simulink model "TST_RailP_VD"  (R2016b)
settings: Solver=FixedStepDiscrete  StartTime=0.0  StopTime=simTime  FixedStep=sampleTime  RelTol=1e-3
values from neighbouring files (symbols this model uses):
  testCase = 1    [initTST_RailP_VD_001.m]    (also in initTST_RailP_VD_002.m = 2)
libraries: simulink x7, UnitTest_Lib x4
settings Model: Creator=liangyunbo  LastModifiedBy=liangyunbo
settings DebuggingCC: SignalRangeChecking=error

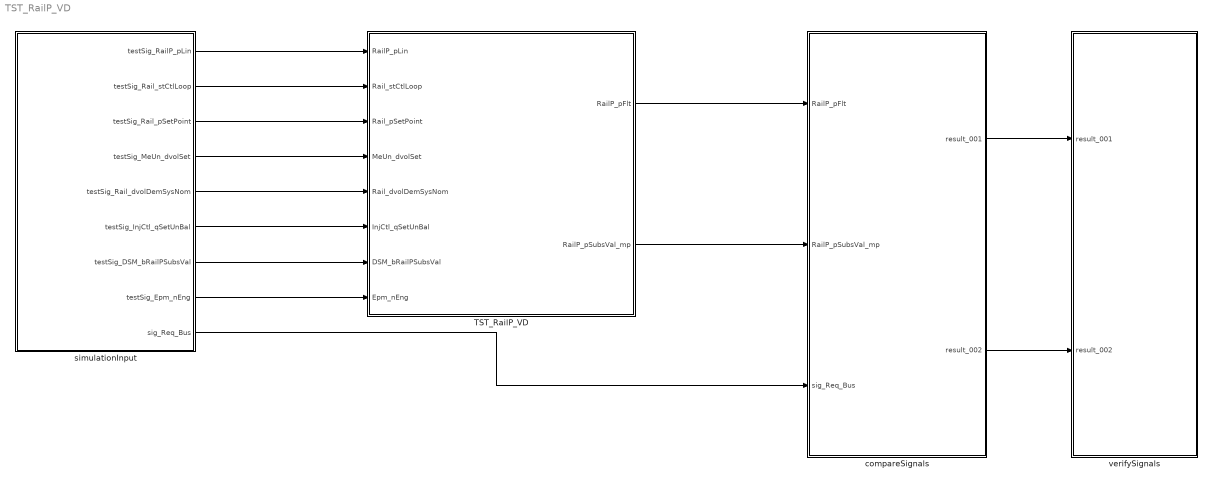
== system TST_RailP_VD ==
  TST_RailP_VD : Subsystem
  compareSignals : Subsystem
  simulationInput : Subsystem
  verifySignals : Subsystem
  wires:
  simulationInput/1(testSig_RailP_pLin) -> TST_RailP_VD/1(RailP_pLin)
  simulationInput/2(testSig_Rail_stCtlLoop) -> TST_RailP_VD/2(Rail_stCtlLoop)
  simulationInput/3(testSig_Rail_pSetPoint) -> TST_RailP_VD/3(Rail_pSetPoint)
  simulationInput/4(testSig_MeUn_dvolSet) -> TST_RailP_VD/4(MeUn_dvolSet)
  simulationInput/5(testSig_Rail_dvolDemSysNom) -> TST_RailP_VD/5(Rail_dvolDemSysNom)
  simulationInput/6(testSig_InjCtl_qSetUnBal) -> TST_RailP_VD/6(InjCtl_qSetUnBal)
  simulationInput/7(testSig_DSM_bRailPSubsVal) -> TST_RailP_VD/7(DSM_bRailPSubsVal)
  simulationInput/8(testSig_Epm_nEng) -> TST_RailP_VD/8(Epm_nEng)
  TST_RailP_VD/1(RailP_pFlt) -> compareSignals/1(RailP_pFlt)
  TST_RailP_VD/2(RailP_pSubsVal_mp) -> compareSignals/2(RailP_pSubsVal_mp)
  simulationInput/9(sig_Req_Bus) -> compareSignals/3(sig_Req_Bus)
  compareSignals/1(result_001) -> verifySignals/1(result_001)
  compareSignals/2(result_002) -> verifySignals/2(result_002)

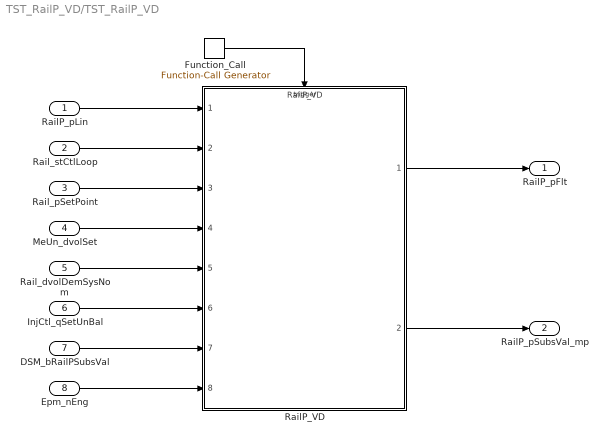
== system TST_RailP_VD/TST_RailP_VD ==
  RailP_pLin : Inport
  Rail_stCtlLoop : Inport  Port=2
  Rail_pSetPoint : Inport  Port=3
  MeUn_dvolSet : Inport  Port=4
  Rail_dvolDemSysNom : Inport  Port=5
  InjCtl_qSetUnBal : Inport  Port=6
  DSM_bRailPSubsVal : Inport  Port=7
  Epm_nEng : Inport  Port=8
  Function_Call : simulink/Ports & Subsystems/Function-Call Generator  sample_time=sampleTime  numberOfIterations=1
  RailP_VD : ModelReference  ModelNameDialog=RailP_VD  SimulationMode=Normal  ModelReferenceVersion=1.40  TriggerPortName=function  TriggerPortTriggerType=function-call  TriggerPortStatesWhenEnabling=held
  RailP_pFlt : Outport
  RailP_pSubsVal_mp : Outport  Port=2
  wires:
  Function_Call/1 -> RailP_VD/Trigger
  RailP_pLin/1 -> RailP_VD/1
  Rail_stCtlLoop/1 -> RailP_VD/2
  Rail_pSetPoint/1 -> RailP_VD/3
  MeUn_dvolSet/1 -> RailP_VD/4
  Rail_dvolDemSysNom/1 -> RailP_VD/5
  InjCtl_qSetUnBal/1 -> RailP_VD/6
  DSM_bRailPSubsVal/1 -> RailP_VD/7
  Epm_nEng/1 -> RailP_VD/8
  RailP_VD/1 -> RailP_pFlt/1
  RailP_VD/2 -> RailP_pSubsVal_mp/1

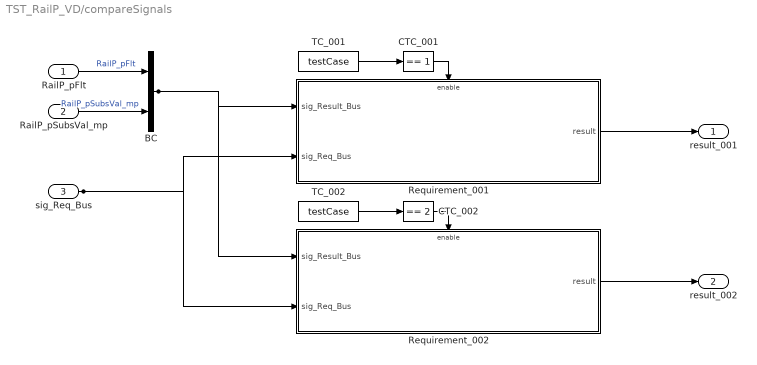
== system TST_RailP_VD/compareSignals ==
  RailP_pFlt : Inport
  RailP_pSubsVal_mp : Inport  Port=2
  sig_Req_Bus : Inport  Port=3
  BC : BusCreator  Inputs=2
  CTC_001 : simulink/Logic and Bit Operations/Compare To Constant  relop===  const=1  OutDataTypeStr=boolean
  CTC_002 : simulink/Logic and Bit Operations/Compare To Constant  relop===  const=2  OutDataTypeStr=boolean
  Requirement_001 : Subsystem
  Requirement_002 : Subsystem
  TC_001 : Constant  Value=testCase
  TC_002 : Constant  Value=testCase
  result_001 : Outport
  result_002 : Outport  Port=2
  wires:
  RailP_pFlt/1 -> BC/1  "RailP_pFlt"
  RailP_pSubsVal_mp/1 -> BC/2  "RailP_pSubsVal_mp"
  TC_001/1 -> CTC_001/1
  CTC_001/1 -> Requirement_001/Enable
  sig_Req_Bus/1 -> Requirement_001/2(sig_Req_Bus), Requirement_002/2(sig_Req_Bus)
  BC/1 -> Requirement_001/1(sig_Result_Bus), Requirement_002/1(sig_Result_Bus)
  Requirement_001/1(result) -> result_001/1
  TC_002/1 -> CTC_002/1
  CTC_002/1 -> Requirement_002/Enable
  Requirement_002/1(result) -> result_002/1

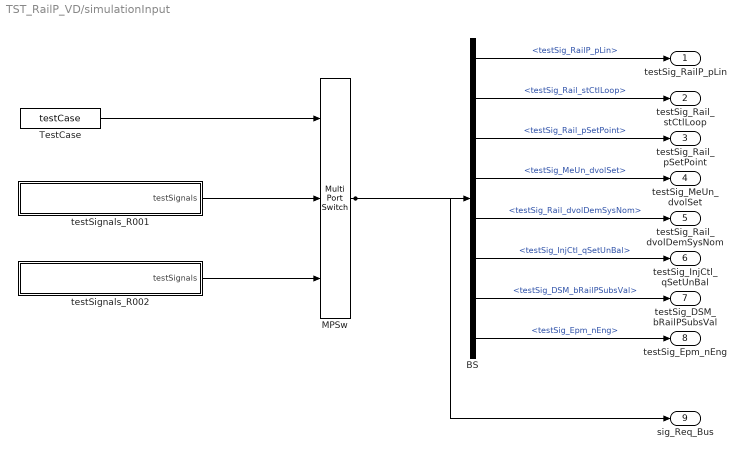
== system TST_RailP_VD/simulationInput ==
  BS : BusSelector  OutputSignals=testSig_RailP_pLin,testSig_Rail_stCtlLoop,testSig_Rail_pSetPoint,testSig_MeUn_dvolSet,testSig_Rail_dvolDemSysNom,testSig_InjCtl_qSetUnBal,testSig_DSM_bRailPSubsVal,testSig_Epm_nEng
  MPSw : MultiPortSwitch  Inputs=2  SaturateOnIntegerOverflow=on  InputSameDT=on
  TestCase : Constant  Value=testCase
  testSignals_R001 : Subsystem
  testSignals_R002 : Subsystem
  testSig_RailP_pLin : Outport
  testSig_Rail_stCtlLoop : Outport  Port=2
  testSig_Rail_pSetPoint : Outport  Port=3
  testSig_MeUn_dvolSet : Outport  Port=4
  testSig_Rail_dvolDemSysNom : Outport  Port=5
  testSig_InjCtl_qSetUnBal : Outport  Port=6
  testSig_DSM_bRailPSubsVal : Outport  Port=7
  testSig_Epm_nEng : Outport  Port=8
  sig_Req_Bus : Outport  Port=9
  wires:
  BS/1 -> testSig_RailP_pLin/1  "<testSig_RailP_pLin>"
  BS/2 -> testSig_Rail_stCtlLoop/1  "<testSig_Rail_stCtlLoop>"
  BS/3 -> testSig_Rail_pSetPoint/1  "<testSig_Rail_pSetPoint>"
  BS/4 -> testSig_MeUn_dvolSet/1  "<testSig_MeUn_dvolSet>"
  BS/5 -> testSig_Rail_dvolDemSysNom/1  "<testSig_Rail_dvolDemSysNom>"
  BS/6 -> testSig_InjCtl_qSetUnBal/1  "<testSig_InjCtl_qSetUnBal>"
  BS/7 -> testSig_DSM_bRailPSubsVal/1  "<testSig_DSM_bRailPSubsVal>"
  BS/8 -> testSig_Epm_nEng/1  "<testSig_Epm_nEng>"
  MPSw/1 -> BS/1, sig_Req_Bus/1
  TestCase/1 -> MPSw/1
  testSignals_R001/1(testSignals) -> MPSw/2
  testSignals_R002/1(testSignals) -> MPSw/3

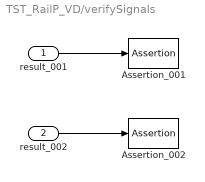
== system TST_RailP_VD/verifySignals ==
  result_001 : Inport
  result_002 : Inport  Port=2
  Assertion_001 : Assertion  Enabled=off
  Assertion_002 : Assertion  Enabled=off
  wires:
  result_001/1 -> Assertion_001/1
  result_002/1 -> Assertion_002/1

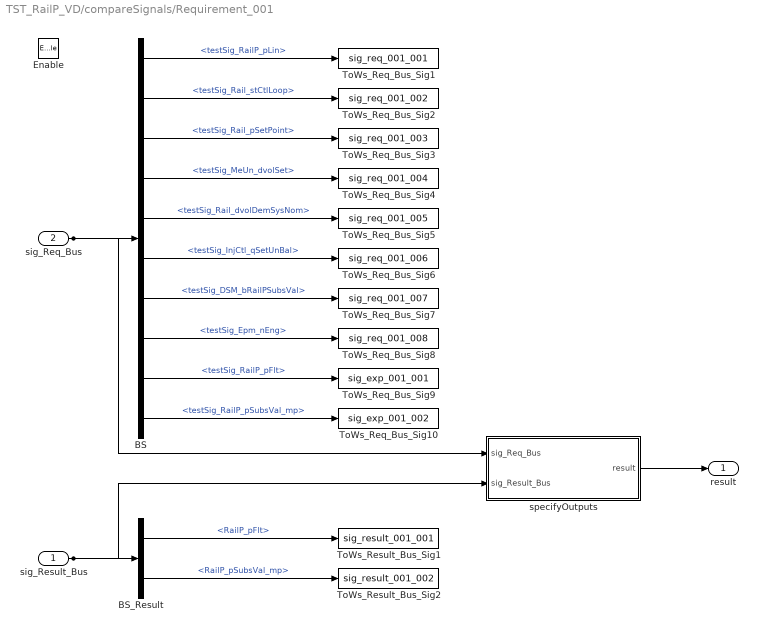
== system TST_RailP_VD/compareSignals/Requirement_001 ==
  sig_Result_Bus : Inport
  sig_Req_Bus : Inport  Port=2
  Enable : EnablePort
  BS : BusSelector  OutputSignals=testSig_RailP_pLin,testSig_Rail_stCtlLoop,testSig_Rail_pSetPoint,testSig_MeUn_dvolSet,testSig_Rail_dvolDemSysNom,testSig_InjCtl_qSetUnBal,testSig_DSM_bRailPSubsVal,testSig_Epm_nEng,testSig_RailP_pFlt,testSig_RailP_pSubsVal_mp
  BS_Result : BusSelector  OutputSignals=RailP_pFlt,RailP_pSubsVal_mp
  ToWs_Req_Bus_Sig1 : ToWorkspace  VariableName=sig_req_001_001  SaveFormat=Structure With Time
  ToWs_Req_Bus_Sig10 : ToWorkspace  VariableName=sig_exp_001_002  SaveFormat=Structure With Time
  ToWs_Req_Bus_Sig2 : ToWorkspace  VariableName=sig_req_001_002  SaveFormat=Structure With Time
  ToWs_Req_Bus_Sig3 : ToWorkspace  VariableName=sig_req_001_003  SaveFormat=Structure With Time
  ToWs_Req_Bus_Sig4 : ToWorkspace  VariableName=sig_req_001_004  SaveFormat=Structure With Time
  ToWs_Req_Bus_Sig5 : ToWorkspace  VariableName=sig_req_001_005  SaveFormat=Structure With Time
  ToWs_Req_Bus_Sig6 : ToWorkspace  VariableName=sig_req_001_006  SaveFormat=Structure With Time
  ToWs_Req_Bus_Sig7 : ToWorkspace  VariableName=sig_req_001_007  SaveFormat=Structure With Time
  ToWs_Req_Bus_Sig8 : ToWorkspace  VariableName=sig_req_001_008  SaveFormat=Structure With Time
  ToWs_Req_Bus_Sig9 : ToWorkspace  VariableName=sig_exp_001_001  SaveFormat=Structure With Time
  ToWs_Result_Bus_Sig1 : ToWorkspace  VariableName=sig_result_001_001  SaveFormat=Structure With Time
  ToWs_Result_Bus_Sig2 : ToWorkspace  VariableName=sig_result_001_002  SaveFormat=Structure With Time
  specifyOutputs : Subsystem
  result : Outport
  wires:
  sig_Req_Bus/1 -> BS/1, specifyOutputs/1(sig_Req_Bus)
  BS/1 -> ToWs_Req_Bus_Sig1/1  "<testSig_RailP_pLin>"
  BS/2 -> ToWs_Req_Bus_Sig2/1  "<testSig_Rail_stCtlLoop>"
  BS/3 -> ToWs_Req_Bus_Sig3/1  "<testSig_Rail_pSetPoint>"
  BS/4 -> ToWs_Req_Bus_Sig4/1  "<testSig_MeUn_dvolSet>"
  BS/5 -> ToWs_Req_Bus_Sig5/1  "<testSig_Rail_dvolDemSysNom>"
  BS/6 -> ToWs_Req_Bus_Sig6/1  "<testSig_InjCtl_qSetUnBal>"
  BS/7 -> ToWs_Req_Bus_Sig7/1  "<testSig_DSM_bRailPSubsVal>"
  BS/8 -> ToWs_Req_Bus_Sig8/1  "<testSig_Epm_nEng>"
  BS/9 -> ToWs_Req_Bus_Sig9/1  "<testSig_RailP_pFlt>"
  BS/10 -> ToWs_Req_Bus_Sig10/1  "<testSig_RailP_pSubsVal_mp>"
  sig_Result_Bus/1 -> BS_Result/1, specifyOutputs/2(sig_Result_Bus)
  BS_Result/1 -> ToWs_Result_Bus_Sig1/1  "<RailP_pFlt>"
  BS_Result/2 -> ToWs_Result_Bus_Sig2/1  "<RailP_pSubsVal_mp>"
  specifyOutputs/1(result) -> result/1

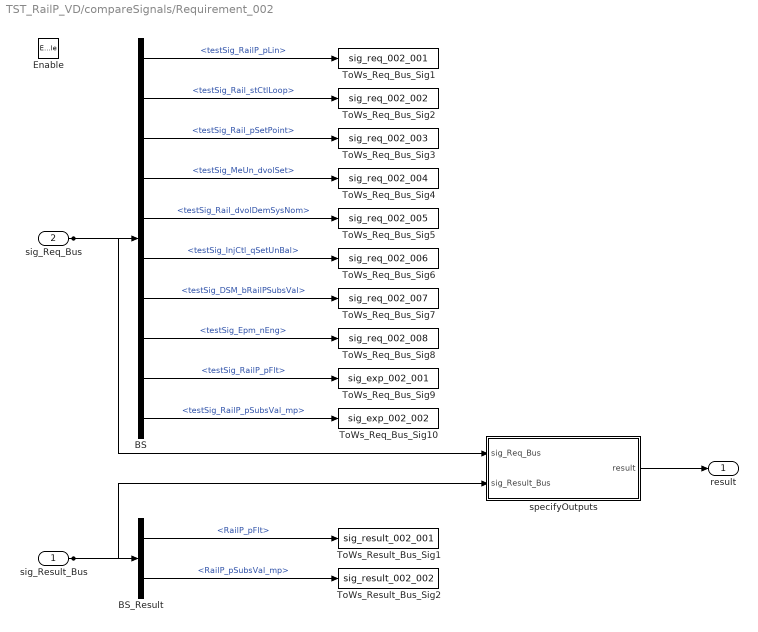
== system TST_RailP_VD/compareSignals/Requirement_002 ==
  sig_Result_Bus : Inport
  sig_Req_Bus : Inport  Port=2
  Enable : EnablePort
  BS : BusSelector  OutputSignals=testSig_RailP_pLin,testSig_Rail_stCtlLoop,testSig_Rail_pSetPoint,testSig_MeUn_dvolSet,testSig_Rail_dvolDemSysNom,testSig_InjCtl_qSetUnBal,testSig_DSM_bRailPSubsVal,testSig_Epm_nEng,testSig_RailP_pFlt,testSig_RailP_pSubsVal_mp
  BS_Result : BusSelector  OutputSignals=RailP_pFlt,RailP_pSubsVal_mp
  ToWs_Req_Bus_Sig1 : ToWorkspace  VariableName=sig_req_002_001  SaveFormat=Structure With Time
  ToWs_Req_Bus_Sig10 : ToWorkspace  VariableName=sig_exp_002_002  SaveFormat=Structure With Time
  ToWs_Req_Bus_Sig2 : ToWorkspace  VariableName=sig_req_002_002  SaveFormat=Structure With Time
  ToWs_Req_Bus_Sig3 : ToWorkspace  VariableName=sig_req_002_003  SaveFormat=Structure With Time
  ToWs_Req_Bus_Sig4 : ToWorkspace  VariableName=sig_req_002_004  SaveFormat=Structure With Time
  ToWs_Req_Bus_Sig5 : ToWorkspace  VariableName=sig_req_002_005  SaveFormat=Structure With Time
  ToWs_Req_Bus_Sig6 : ToWorkspace  VariableName=sig_req_002_006  SaveFormat=Structure With Time
  ToWs_Req_Bus_Sig7 : ToWorkspace  VariableName=sig_req_002_007  SaveFormat=Structure With Time
  ToWs_Req_Bus_Sig8 : ToWorkspace  VariableName=sig_req_002_008  SaveFormat=Structure With Time
  ToWs_Req_Bus_Sig9 : ToWorkspace  VariableName=sig_exp_002_001  SaveFormat=Structure With Time
  ToWs_Result_Bus_Sig1 : ToWorkspace  VariableName=sig_result_002_001  SaveFormat=Structure With Time
  ToWs_Result_Bus_Sig2 : ToWorkspace  VariableName=sig_result_002_002  SaveFormat=Structure With Time
  specifyOutputs : Subsystem
  result : Outport
  wires:
  sig_Req_Bus/1 -> BS/1, specifyOutputs/1(sig_Req_Bus)
  BS/1 -> ToWs_Req_Bus_Sig1/1  "<testSig_RailP_pLin>"
  BS/2 -> ToWs_Req_Bus_Sig2/1  "<testSig_Rail_stCtlLoop>"
  BS/3 -> ToWs_Req_Bus_Sig3/1  "<testSig_Rail_pSetPoint>"
  BS/4 -> ToWs_Req_Bus_Sig4/1  "<testSig_MeUn_dvolSet>"
  BS/5 -> ToWs_Req_Bus_Sig5/1  "<testSig_Rail_dvolDemSysNom>"
  BS/6 -> ToWs_Req_Bus_Sig6/1  "<testSig_InjCtl_qSetUnBal>"
  BS/7 -> ToWs_Req_Bus_Sig7/1  "<testSig_DSM_bRailPSubsVal>"
  BS/8 -> ToWs_Req_Bus_Sig8/1  "<testSig_Epm_nEng>"
  BS/9 -> ToWs_Req_Bus_Sig9/1  "<testSig_RailP_pFlt>"
  BS/10 -> ToWs_Req_Bus_Sig10/1  "<testSig_RailP_pSubsVal_mp>"
  sig_Result_Bus/1 -> BS_Result/1, specifyOutputs/2(sig_Result_Bus)
  BS_Result/1 -> ToWs_Result_Bus_Sig1/1  "<RailP_pFlt>"
  BS_Result/2 -> ToWs_Result_Bus_Sig2/1  "<RailP_pSubsVal_mp>"
  specifyOutputs/1(result) -> result/1

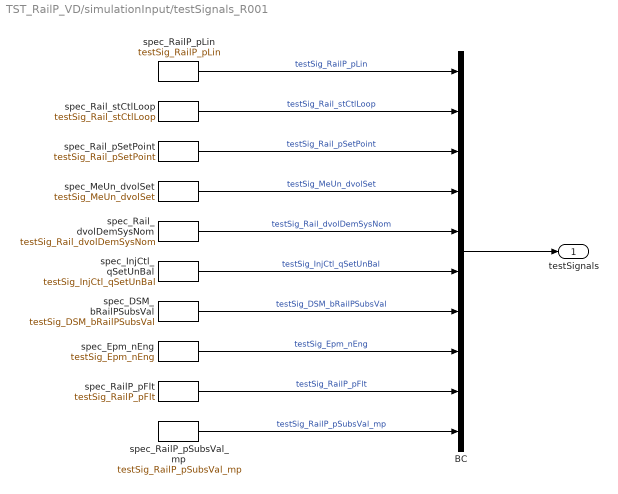
== system TST_RailP_VD/simulationInput/testSignals_R001 ==
  BC : BusCreator  Inputs=10
  spec_DSM_bRailPSubsVal : FromWorkspace  VariableName=testSig_DSM_bRailPSubsVal  Interpolate=off  OutputAfterFinalValue=Holding final value
  spec_Epm_nEng : FromWorkspace  VariableName=testSig_Epm_nEng  Interpolate=off  OutputAfterFinalValue=Holding final value
  spec_InjCtl_qSetUnBal : FromWorkspace  VariableName=testSig_InjCtl_qSetUnBal  Interpolate=off  OutputAfterFinalValue=Holding final value
  spec_MeUn_dvolSet : FromWorkspace  VariableName=testSig_MeUn_dvolSet  Interpolate=off  OutputAfterFinalValue=Holding final value
  spec_RailP_pFlt : FromWorkspace  VariableName=testSig_RailP_pFlt  Interpolate=off  OutputAfterFinalValue=Holding final value
  spec_RailP_pLin : FromWorkspace  VariableName=testSig_RailP_pLin  Interpolate=off  OutputAfterFinalValue=Holding final value
  spec_RailP_pSubsVal_mp : FromWorkspace  VariableName=testSig_RailP_pSubsVal_mp  Interpolate=off  OutputAfterFinalValue=Holding final value
  spec_Rail_dvolDemSysNom : FromWorkspace  VariableName=testSig_Rail_dvolDemSysNom  Interpolate=off  OutputAfterFinalValue=Holding final value
  spec_Rail_pSetPoint : FromWorkspace  VariableName=testSig_Rail_pSetPoint  Interpolate=off  OutputAfterFinalValue=Holding final value
  spec_Rail_stCtlLoop : FromWorkspace  VariableName=testSig_Rail_stCtlLoop  Interpolate=off  OutputAfterFinalValue=Holding final value
  testSignals : Outport
  wires:
  BC/1 -> testSignals/1
  spec_RailP_pLin/1 -> BC/1  "testSig_RailP_pLin"
  spec_Rail_stCtlLoop/1 -> BC/2  "testSig_Rail_stCtlLoop"
  spec_Rail_pSetPoint/1 -> BC/3  "testSig_Rail_pSetPoint"
  spec_MeUn_dvolSet/1 -> BC/4  "testSig_MeUn_dvolSet"
  spec_Rail_dvolDemSysNom/1 -> BC/5  "testSig_Rail_dvolDemSysNom"
  spec_InjCtl_qSetUnBal/1 -> BC/6  "testSig_InjCtl_qSetUnBal"
  spec_DSM_bRailPSubsVal/1 -> BC/7  "testSig_DSM_bRailPSubsVal"
  spec_Epm_nEng/1 -> BC/8  "testSig_Epm_nEng"
  spec_RailP_pFlt/1 -> BC/9  "testSig_RailP_pFlt"
  spec_RailP_pSubsVal_mp/1 -> BC/10  "testSig_RailP_pSubsVal_mp"

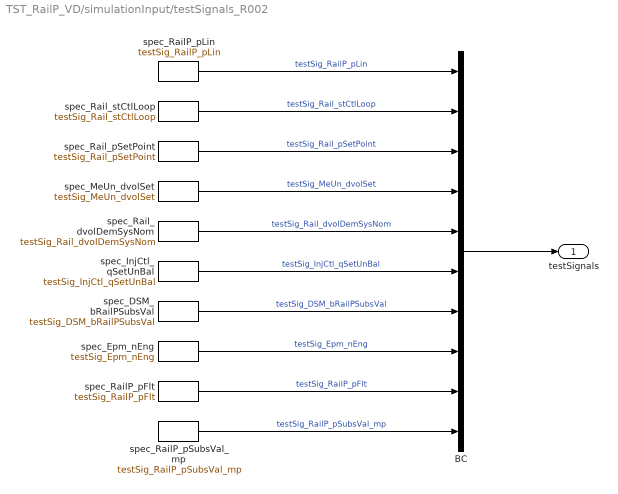
== system TST_RailP_VD/simulationInput/testSignals_R002 ==
  BC : BusCreator  Inputs=10
  spec_DSM_bRailPSubsVal : FromWorkspace  VariableName=testSig_DSM_bRailPSubsVal  Interpolate=off  OutputAfterFinalValue=Holding final value
  spec_Epm_nEng : FromWorkspace  VariableName=testSig_Epm_nEng  Interpolate=off  OutputAfterFinalValue=Holding final value
  spec_InjCtl_qSetUnBal : FromWorkspace  VariableName=testSig_InjCtl_qSetUnBal  Interpolate=off  OutputAfterFinalValue=Holding final value
  spec_MeUn_dvolSet : FromWorkspace  VariableName=testSig_MeUn_dvolSet  Interpolate=off  OutputAfterFinalValue=Holding final value
  spec_RailP_pFlt : FromWorkspace  VariableName=testSig_RailP_pFlt  Interpolate=off  OutputAfterFinalValue=Holding final value
  spec_RailP_pLin : FromWorkspace  VariableName=testSig_RailP_pLin  Interpolate=off  OutputAfterFinalValue=Holding final value
  spec_RailP_pSubsVal_mp : FromWorkspace  VariableName=testSig_RailP_pSubsVal_mp  Interpolate=off  OutputAfterFinalValue=Holding final value
  spec_Rail_dvolDemSysNom : FromWorkspace  VariableName=testSig_Rail_dvolDemSysNom  Interpolate=off  OutputAfterFinalValue=Holding final value
  spec_Rail_pSetPoint : FromWorkspace  VariableName=testSig_Rail_pSetPoint  Interpolate=off  OutputAfterFinalValue=Holding final value
  spec_Rail_stCtlLoop : FromWorkspace  VariableName=testSig_Rail_stCtlLoop  Interpolate=off  OutputAfterFinalValue=Holding final value
  testSignals : Outport
  wires:
  BC/1 -> testSignals/1
  spec_RailP_pLin/1 -> BC/1  "testSig_RailP_pLin"
  spec_Rail_stCtlLoop/1 -> BC/2  "testSig_Rail_stCtlLoop"
  spec_Rail_pSetPoint/1 -> BC/3  "testSig_Rail_pSetPoint"
  spec_MeUn_dvolSet/1 -> BC/4  "testSig_MeUn_dvolSet"
  spec_Rail_dvolDemSysNom/1 -> BC/5  "testSig_Rail_dvolDemSysNom"
  spec_InjCtl_qSetUnBal/1 -> BC/6  "testSig_InjCtl_qSetUnBal"
  spec_DSM_bRailPSubsVal/1 -> BC/7  "testSig_DSM_bRailPSubsVal"
  spec_Epm_nEng/1 -> BC/8  "testSig_Epm_nEng"
  spec_RailP_pFlt/1 -> BC/9  "testSig_RailP_pFlt"
  spec_RailP_pSubsVal_mp/1 -> BC/10  "testSig_RailP_pSubsVal_mp"

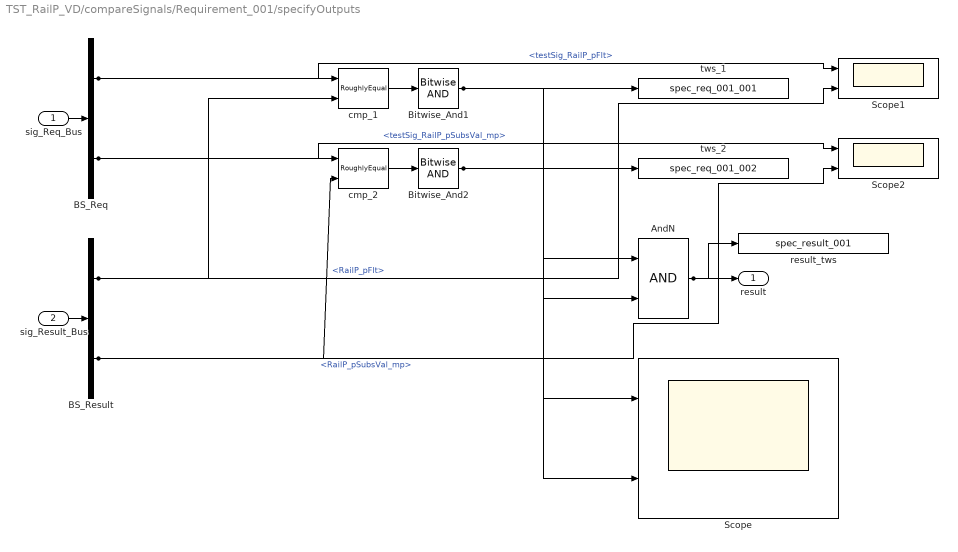
== system TST_RailP_VD/compareSignals/Requirement_001/specifyOutputs ==
  sig_Req_Bus : Inport
  sig_Result_Bus : Inport  Port=2
  AndN : Logic
  BS_Req : BusSelector  OutputSignals=testSig_RailP_pFlt,testSig_RailP_pSubsVal_mp
  BS_Result : BusSelector  OutputSignals=RailP_pFlt,RailP_pSubsVal_mp
  Bitwise_And1 : simulink/Logic and Bit Operations/Bitwise Operator  logicop=AND  UseBitMask=off  BitMask=bin2dec('11011001')  BitMaskRealWorld=Stored Integer
  Bitwise_And2 : simulink/Logic and Bit Operations/Bitwise Operator  logicop=AND  UseBitMask=off  BitMask=bin2dec('11011001')  BitMaskRealWorld=Stored Integer
  Scope : Scope  NumInputPorts=2
  Scope1 : Scope  NumInputPorts=2
  Scope2 : Scope  NumInputPorts=2
  cmp_1 : UnitTest_Lib/RoughlyEqual  slope=0.1
  cmp_2 : UnitTest_Lib/RoughlyEqual  slope=0.1
  result_tws : ToWorkspace  VariableName=spec_result_001
  tws_1 : ToWorkspace  VariableName=spec_req_001_001
  tws_2 : ToWorkspace  VariableName=spec_req_001_002
  result : Outport
  wires:
  sig_Req_Bus/1 -> BS_Req/1
  sig_Result_Bus/1 -> BS_Result/1
  AndN/1 -> result/1, result_tws/1
  BS_Req/1 -> cmp_1/1, Scope1/1  "<testSig_RailP_pFlt>"
  BS_Result/1 -> cmp_1/2, Scope1/2  "<RailP_pFlt>"
  cmp_1/1 -> Bitwise_And1/1
  Bitwise_And1/1 -> tws_1/1, AndN/1, Scope/1
  BS_Req/2 -> cmp_2/1, Scope2/1  "<testSig_RailP_pSubsVal_mp>"
  BS_Result/2 -> cmp_2/2, Scope2/2  "<RailP_pSubsVal_mp>"
  cmp_2/1 -> Bitwise_And2/1
  Bitwise_And2/1 -> tws_2/1, AndN/2, Scope/2

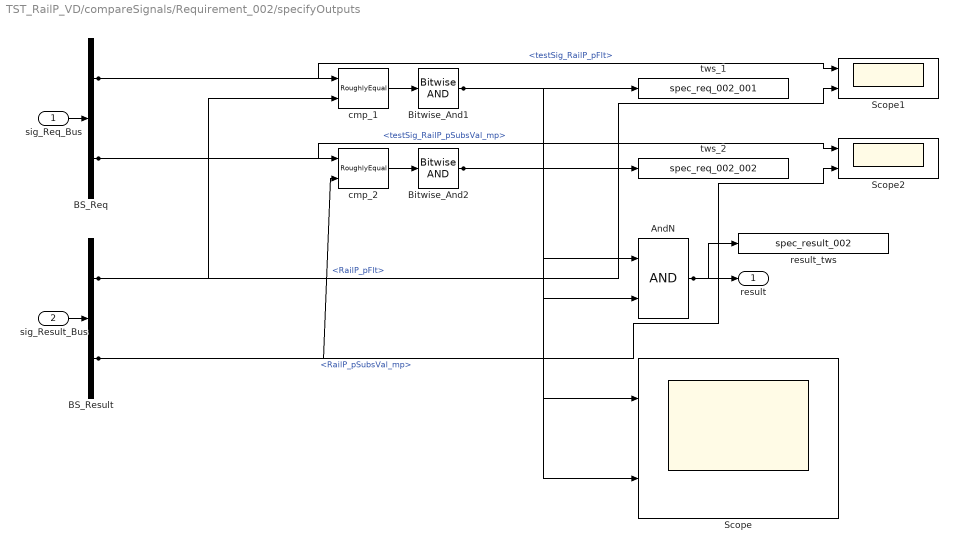
== system TST_RailP_VD/compareSignals/Requirement_002/specifyOutputs ==
  sig_Req_Bus : Inport
  sig_Result_Bus : Inport  Port=2
  AndN : Logic
  BS_Req : BusSelector  OutputSignals=testSig_RailP_pFlt,testSig_RailP_pSubsVal_mp
  BS_Result : BusSelector  OutputSignals=RailP_pFlt,RailP_pSubsVal_mp
  Bitwise_And1 : simulink/Logic and Bit Operations/Bitwise Operator  logicop=AND  UseBitMask=off  BitMask=bin2dec('11011001')  BitMaskRealWorld=Stored Integer
  Bitwise_And2 : simulink/Logic and Bit Operations/Bitwise Operator  logicop=AND  UseBitMask=off  BitMask=bin2dec('11011001')  BitMaskRealWorld=Stored Integer
  Scope : Scope  NumInputPorts=2
  Scope1 : Scope  NumInputPorts=2
  Scope2 : Scope  NumInputPorts=2
  cmp_1 : UnitTest_Lib/RoughlyEqual  slope=0.1
  cmp_2 : UnitTest_Lib/RoughlyEqual  slope=0.1
  result_tws : ToWorkspace  VariableName=spec_result_002
  tws_1 : ToWorkspace  VariableName=spec_req_002_001
  tws_2 : ToWorkspace  VariableName=spec_req_002_002
  result : Outport
  wires:
  sig_Req_Bus/1 -> BS_Req/1
  sig_Result_Bus/1 -> BS_Result/1
  AndN/1 -> result/1, result_tws/1
  BS_Req/1 -> cmp_1/1, Scope1/1  "<testSig_RailP_pFlt>"
  BS_Result/1 -> cmp_1/2, Scope1/2  "<RailP_pFlt>"
  cmp_1/1 -> Bitwise_And1/1
  Bitwise_And1/1 -> tws_1/1, AndN/1, Scope/1
  BS_Req/2 -> cmp_2/1, Scope2/1  "<testSig_RailP_pSubsVal_mp>"
  BS_Result/2 -> cmp_2/2, Scope2/2  "<RailP_pSubsVal_mp>"
  cmp_2/1 -> Bitwise_And2/1
  Bitwise_And2/1 -> tws_2/1, AndN/2, Scope/2
